simulink model "experimenteren"  (R2013a)
settings: Solver=FixedStepDiscrete  StartTime=0.0  StopTime=10  FixedStep=1/44100  RelTol=1e-3
InitFcn:
  | input_frame_size = 4096;
  | frame_size = 4096;
  | overlap = 0.5;
  | alpha = 1.5;
  | 
  | k = round(frame_size - alpha*(1-overlap)*frame_size);
libraries: dspmtrx3 x5, dspsigops x1, dspvision x1
settings Model: Creator=Tomas  LastModifiedBy=Tomas

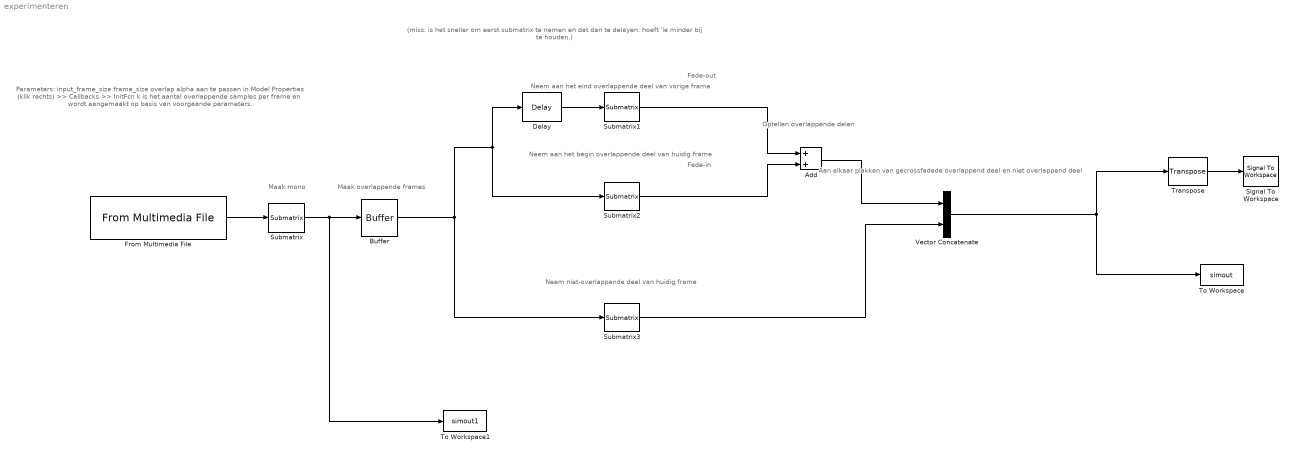
== system experimenteren ==
  note: (miss. is het sneller om eerst submatrix te nemen
      | en dat dan te delayen: hoeft 'ie minder bij te houden.)
  note: Aan elkaar plakken van
      | gecrossfadede overlappend deel
      | en niet overlappend deel
  note: Optellen
      | overlappende delen
  note: Neem niet-overlappende deel
      | van huidig frame
  note: Fade-in
  note: Fade-out
  note: Neem aan het begin overlappende
      | deel van huidig frame
  note: Neem aan het eind overlappende
      | deel van vorige frame
  note: Parameters:
      | input_frame_size
      | frame_size
      | overlap
      | alpha
      |
      | aan te passen in
      |
      | Model Properties (klik rechts)
      |  >> Callbacks >> InitFcn
      |
      | k is het aantal overlappende
      |  samples per frame en wordt
      | aangemaakt op basis van
      | voorgaande parameters.
  note: Maak overlappende frames
  note: Maak mono
  Add : Sum  Inputs=2
  Buffer : Buffer  N=frame_size  V=round(frame_size*overlap)  TreatMby1Signals=One channel
  Delay : dspsigops/Delay  InputProcessing=Columns as channels (frame based)  dly_unit=Frames  delay=1  ic_detail=off  dif_ic_for_ch=off  dif_ic_for_dly=off  ic=0  reset_popup=None
  From Multimedia File : dspvision/From Multimedia File  inputFilename=D:\Dropbox\P&O3 - Time Scaling 2013\van_jszurleys_ftp\Speech materials\goedele1.wav  loop=on  numPlays=1  outputStreams=Audio only  videoDataType=single  audioDataType=double  inheritSampleTime=on  userDefinedSampleTime=1/30  noAudioOutput=off  isIntensityVideo=off  fourcc=RGB  colorVideoFormat=Separate color signals  outputEOF=off  dataOrg=Column-major  audioFrameSize=input_frame_size  computeAudioFrameSize=off  outSamplingMode=Frame based
  Signal To Workspace : SignalToWorkspace  VariableName=yout
      settings: CopyFcn=dspblkcopystw(gcbh);
  Submatrix : dspmtrx3/Submatrix  RowSpan=All rows  RowStartMode=First  RowStartIndex=1  RowEndMode=Last  RowEndIndex=1  ColSpan=One column  ColStartMode=First  ColStartIndex=1  ColEndMode=Last  ColEndIndex=1
  Submatrix1 : dspmtrx3/Submatrix  RowSpan=Range of rows  RowStartMode=Offset from last  RowStartIndex=k-1  RowEndMode=Last  RowEndIndex=1  ColSpan=All columns  ColStartMode=Offset from last  ColStartIndex=k  ColEndMode=Last  ColEndIndex=1
  Submatrix2 : dspmtrx3/Submatrix  RowSpan=Range of rows  RowStartMode=First  RowStartIndex=1  RowEndMode=Index  RowEndIndex=k  ColSpan=All columns  ColStartMode=Offset from last  ColStartIndex=k  ColEndMode=Last  ColEndIndex=1
  Submatrix3 : dspmtrx3/Submatrix  RowSpan=Range of rows  RowStartMode=Index  RowStartIndex=k+1  RowEndMode=Offset from last  RowEndIndex=k  ColSpan=All columns  ColStartMode=Offset from last  ColStartIndex=k  ColEndMode=Last  ColEndIndex=1
  To Workspace : ToWorkspace  VariableName=simout  SampleTime=-1
  To Workspace1 : ToWorkspace  VariableName=simout1  SampleTime=-1
  Transpose : dspmtrx3/Transpose  Hermitian=off  overflowFlag=off
  Vector Concatenate : Concatenate  Mode=Multidimensional array
  wires:
  From Multimedia File/1 -> Submatrix/1
  Submatrix/1 -> Buffer/1, To Workspace1/1
  Transpose/1 -> Signal To Workspace/1
  Buffer/1 -> Submatrix2/1, Delay/1, Submatrix3/1
  Delay/1 -> Submatrix1/1
  Add/1 -> Vector Concatenate/1
  Submatrix3/1 -> Vector Concatenate/2
  Vector Concatenate/1 -> Transpose/1, To Workspace/1
  Submatrix2/1 -> Add/2
  Submatrix1/1 -> Add/1
